simulink model "constantTorqueDemo"  (Simulink 7.6)
settings: Solver=ode45  StartTime=0.0  StopTime=inf  RelTol=1e-3
undefined symbols (not defined in the file or in its folder): PendulumPlant, PendulumVisualizer
libraries: robotlib x3, simulink x2
settings Model: Creator=russt  LastModifiedBy=russt

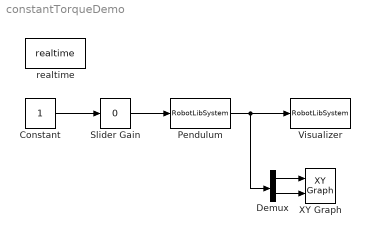
== system constantTorqueDemo ==
  Constant : Constant
  Demux : Demux  Outputs=2
  Pendulum : robotlib/RobotLibSystem  sysobj=PendulumPlant()
  Slider Gain : simulink/Math Operations/Slider Gain  SystemSampleTime=-1  low=-5  gain=0  high=5
  Visualizer : robotlib/RobotLibSystem  sysobj=PendulumVisualizer()
  XY Graph : simulink/Sinks/XY Graph  SystemSampleTime=-1  xmin=-pi  xmax=pi  ymin=-4  ymax=4  st=-1
  realtime : robotlib/realtime  sample_time=.1
  wires:
  Pendulum/1 -> Visualizer/1, Demux/1
  Slider Gain/1 -> Pendulum/1
  Constant/1 -> Slider Gain/1
  Demux/1 -> XY Graph/1
  Demux/2 -> XY Graph/2
